simulink model "mcb_pmsm_sixstep_hall_dsPIC33CK256MP508"  (R2022a)
settings: Solver=FixedStepDiscrete  StartTime=0.0  StopTime=12  FixedStep=.00005  RelTol=1e-3  EnableMultiTasking=on
PreLoadFcn:
  | mcb_pmsm_sixstep_hall_lvmc_data;
InitFcn:
  | mcb_pmsm_sixstep_hall_lvmc_data;
values from neighbouring files (symbols this model uses):
  PI_params = mcb.internal.SetControllerParameters(bldc,inverter,PU_System,T_pwm,Ts,Ts_speed)    [mcb_bldc_sixstep_hall_lvmc_data.m]    (also in mcb_pmsm_sixstep_hall_lvmc_data.m)
  PU_System = mcb_SetPUSystem(bldc,inverter)    [mcb_bldc_sixstep_hall_lvmc_data.m]    (also in mcb_pmsm_sixstep_hall_lvmc_data.m)
  PWM_frequency = 20e3    (= 20000)    [mcb_bldc_sixstep_hall_lvmc_data.m]    (also in mcb_pmsm_sixstep_hall_lvmc_data.m)
  Ts = T_pwm    (= 5e-05)    [mcb_bldc_sixstep_hall_lvmc_data.m]    (also in mcb_pmsm_sixstep_hall_lvmc_data.m)
  Ts_speed = 30*Ts    (= 0.0015)    [mcb_bldc_sixstep_hall_lvmc_data.m]    (also in mcb_pmsm_sixstep_hall_lvmc_data.m)
undefined symbols (not defined in the file or in its folder): A0, AN0, AN1, B0, B2, bldc, C9, D13, inverter, MaxPer, ms, P32, P57, P77, Pin, pmsm, PWM1max, Resol, s, us
libraries: MCHP_Blockset x22, nesl_utility x14, simulink x12, fl_lib x9, ee_lib x5, mcbcontrolslib x4, mcbpositiondecoderlib x2, slpidlib x1
(part 1 of 3)
settings Model: Creator=M91449  LastModifiedBy=I52209
settings SolverCC: AlgebraicLoopSolver=TrustRegion
settings DataIOCC: LimitDataPoints=on  ReturnWorkspaceOutputs=off
settings OptimizationCC: DefaultParameterBehavior=Inlined  InlineInvariantSignals=on  LifeSpan=1  EfficientTunableParamExpr=on
settings DebuggingCC: MultiTaskDSMMsg=none  UnconnectedInputMsg=warning  UnconnectedOutputMsg=warning  UnconnectedLineMsg=warning  SFUnexpectedBacktrackingDiag=warning  SFNoUnconditionalDefaultTransitionDiag=warning  SFExecutionAtInitializationDiag=none  SFMachineParentedDataDiag=warning  ArithmeticOperatorsInVariantConditions=warning
settings HardwareCC: ProdBitPerInt=16  ProdBitPerPointer=16  ProdBitPerSizeT=16  ProdBitPerPtrDiffT=16  ProdLargestAtomicInteger=Integer  ProdLargestAtomicFloat=None  ProdWordSize=16  ProdHWDeviceType=Generic->Custom
settings ModelReferenceCC: ModelReferenceNumInstancesAllowed=Single  PropagateSignalLabelsOutOfModel=off
settings SFSimCC: SimUseLocalCustomCode=off  MATLABDynamicMemAlloc=off  CustomCodeUndefinedFunction=UseInterfaceOnly
settings RTWCC: Description=Microchip Embedded Target PIC24 dsPIC30 dsPIC33 (real-time)  SystemTargetFile=MCHP_dsPIC_stf.tlc  TemplateMakefile=MCHP_dsPIC.tmf  RTWUseLocalCustomCode=off  CustomInclude=/Clib  CustomSource=function.c  IncludeHyperlinkInReport=on  GenerateCodeMetricsReport=on  DLArmComputeVersion=19.05
settings CodeAppCC: IgnoreCustomStorageClasses=off  MaxIdLength=255  StateflowObjectComments=on
settings STFCustomTargetCC: TargetLibSuffix=_lib.a  CodeReplacementLibrary=Microchip Code Replacement Library for dsPIC  CombineOutputUpdateFcns=on  ERTCustomFileBanners=on  SupportContinuousTime=off  RemoveResetFunc=on  MATLABClassNameForMDSCustomization=Simulink.SoftwareTarget.ERTCustomization  GRTInterface=off  SystemTargetFile=MCHP_dsPIC_stf.tlc
settings ERTTargetCC: TargetLibSuffix=_lib.a  CodeReplacementLibrary=Microchip Code Replacement Library for dsPIC  MultiwordLength=2048  ParMdlRefBuildCompliant=off  CompOptLevelCompliant=off  ConcurrentExecutionCompliant=off  SupportNonInlinedSFcns=on  ModelStepFunctionPrototypeControlCompliant=off  CPPClassGenCompliant=off  UseToolchainInfoCompliant=off  InlinedParameterPlacement=NonHierarchical  ERTSrcFileBannerTemplate=MCHP_dsPIC_code_template.cgt  ERTHdrFileBannerTemplate=MCHP_dsPIC_code_template.cgt  ERTDataSrcFileTemplate=MCHP_dsPIC_code_template.cgt  ERTDataHdrFileTemplate=MCHP_dsPIC_code_template.cgt  ERTCustomFileTemplate=MCHP_main.tlc  ConvertIfToSwitch=off  SuppressUnreachableDefaultCases=off
settings ConfigComp: CovMetricSettings=dw  CovSaveCumulativeToWorkspaceVar=on  CovSaveSingleToWorkspaceVar=on  CovExternalEMLEnable=off

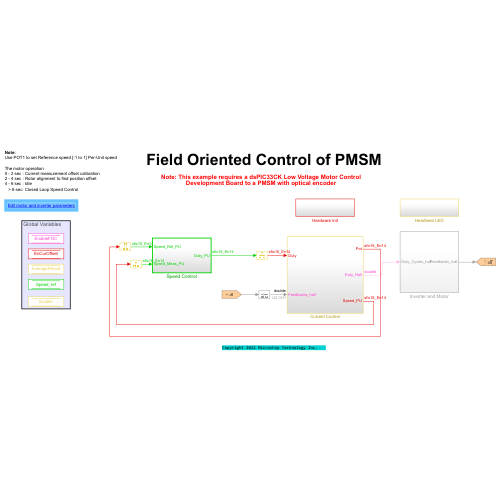
[thumbnail: Simulink's stored preview of the top-level diagram]
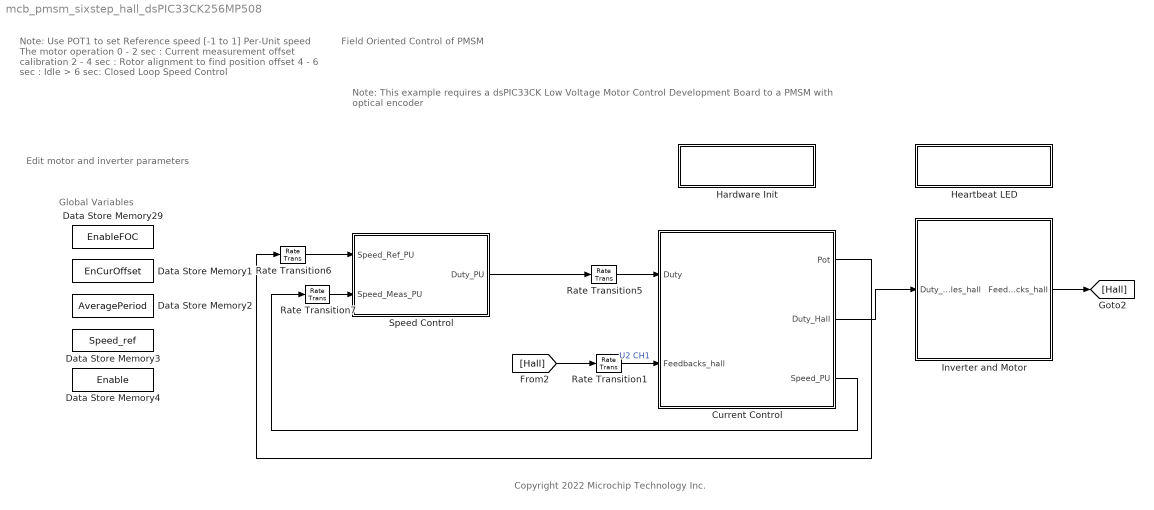
== system mcb_pmsm_sixstep_hall_dsPIC33CK256MP508 ==
  note: Edit motor and inverter parameters
  note: Note:
      | Use POT1 to set Reference speed [-1 to 1] Per-Unit speed
      |
      | The motor operation
      | 0 - 2 sec : Current measurement offset calibration
      | 2 - 4 sec : Rotor alignment to find position offset
      | 4 - 6 sec : Idle
      | > 6 sec: Closed Loop Speed Control
  note: Global Variables
  note: Field Oriented Control of PMSM
  note: Note: This example requires a dsPIC33CK Low Voltage Motor Control Development Board to a PMSM with optical encoder
  note: Copyright 2022 Microchip Technology Inc.
  Current Control : Subsystem  VariantControl=Optimized
  Data Store Memory1 : DataStoreMemory  DataStoreName=EnCurOffset  ShowAdditionalParam=off  OutDataTypeStr=boolean
  Data Store Memory2 : DataStoreMemory  DataStoreName=AveragePeriod  ShowAdditionalParam=off  OutDataTypeStr=uint16
  Data Store Memory29 : DataStoreMemory  DataStoreName=EnableFOC  ShowAdditionalParam=off  OutDataTypeStr=boolean
  Data Store Memory3 : DataStoreMemory  DataStoreName=Speed_ref  ShowAdditionalParam=off  OutDataTypeStr=dataType
  Data Store Memory4 : DataStoreMemory  DataStoreName=Enable  ShowAdditionalParam=off  OutDataTypeStr=boolean
  Hardware Init : Subsystem
  Heartbeat LED : Subsystem
  Inverter and Motor : Subsystem
  Rate Transition{1,5..7} (4 alike) : RateTransition  Deterministic=off
  Speed Control : Subsystem  TreatAsAtomicUnit=on  SystemSampleTime=Ts_speed
  wires:
  Rate Transition6/1 -> Speed Control/1(Speed_Ref_PU)
  Rate Transition7/1 -> Speed Control/2(Speed_Meas_PU)
  Speed Control/1(Duty_PU) -> Rate Transition5/1
  Rate Transition5/1 -> Current Control/1(Duty)
  Current Control/1(Pot) -> Rate Transition6/1
  Rate Transition1/1 -> Current Control/2(Feedbacks_hall)  "U2 CH1"
  Inverter and Motor/1(Feedbacks_hall) -> [Hall]
  [Hall] -> Rate Transition1/1
  Current Control/2(Duty_Hall) -> Inverter and Motor/1(Duty_Cycles_hall)
  Current Control/3(Speed_PU) -> Rate Transition7/1

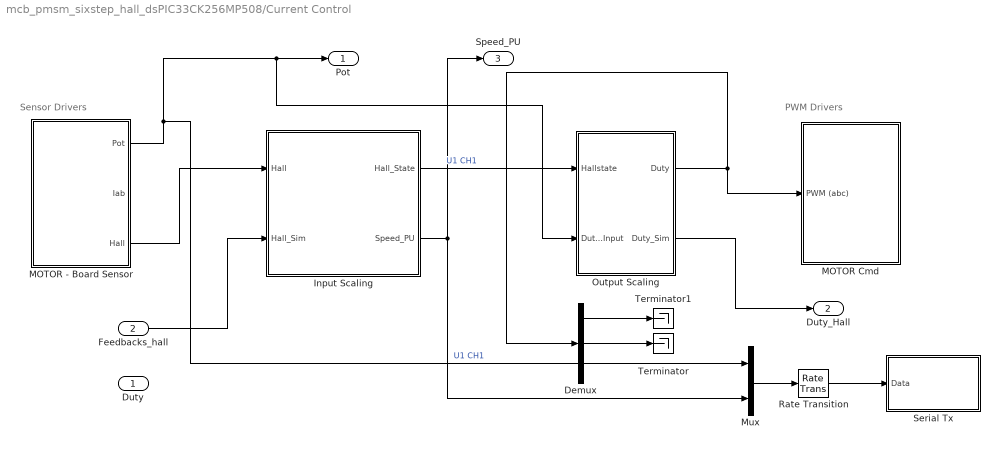
== system mcb_pmsm_sixstep_hall_dsPIC33CK256MP508/Current Control ==
  note: Sensor Drivers
  note: PWM Drivers
  Duty : Inport
  Feedbacks_hall : Inport  Port=2
  Demux : Demux  Outputs=3
  Input Scaling : Subsystem
  MOTOR Cmd : Subsystem
  MOTOR - Board Sensor : Subsystem
  Mux : Mux  Inputs=2
  Output Scaling : Subsystem
  Rate Transition : RateTransition  Integrity=off  Deterministic=off  OutPortSampleTime=Ts*100
  Serial Tx : Subsystem
  Terminator : Terminator
  Terminator1 : Terminator
  Pot : Outport
  Duty_Hall : Outport  Port=2
  Speed_PU : Outport  Port=3
  wires:
  Rate Transition/1 -> Serial Tx/1(Data)
  Mux/1 -> Rate Transition/1
  Feedbacks_hall/1 -> Input Scaling/2(Hall_Sim)
  Input Scaling/1(Hall_State) -> Output Scaling/1(Hallstate)  "U1 CH1"
  Output Scaling/1(Duty) -> MOTOR Cmd/1(PWM (abc)), Demux/1
  Output Scaling/2(Duty_Sim) -> Duty_Hall/1
  Demux/2 -> Terminator/1
  Demux/1 -> Terminator1/1
  MOTOR - Board Sensor/1(Pot) -> Mux/1, Output Scaling/2(Duty_Input), Pot/1  "U1 CH1"
  Input Scaling/2(Speed_PU) -> Mux/2, Speed_PU/1
  MOTOR - Board Sensor/3(Hall) -> Input Scaling/1(Hall)

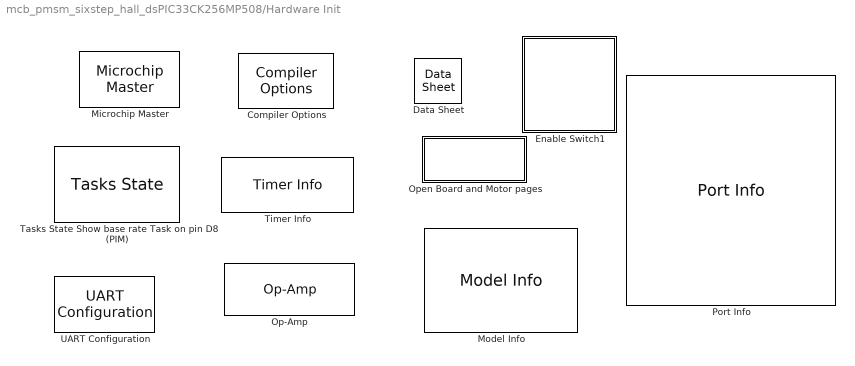
== system mcb_pmsm_sixstep_hall_dsPIC33CK256MP508/Hardware Init ==
  Compiler Options : MCHP_Blockset/System Configuration/Compiler Options  Priority=1  LATEST_CMPLR=on  COMP_LIST=Dynamic Options  COMP_LIST_TXT=xc16 - v1.70  DFP_LIST=Dynamic Options  DFP_LIST_TXT=v 1.7.208  CMSIS_DSP=Dynamic Options  CMSIS_DSP_TXT=Dynamic Options  USE_64BIT_DOUBLE=off  MCHP_MULTITHREAD_COMPILATION=on  UseCustom_LinkerScript=off  MCHP_MASTERLINK=mcb_pmsm_sixstep_hall_dsPIC33CK256MP508/Hardware Init/Microchip Master  OPTIMIZATION_LEVEL=3  MPLAB_LINKLIB=default  MPLAB_LINKLIB1=default  CodeReplacement=Dynamic Options  CodeReplacement_TXT=Microchip Code Replacement Library for dsPIC  OPTIMIZATION_FLTO=on  OPTIMIZATION_REORDER=off  UNROLL_LOOPS=on  PROCEDURAL_ABSTRACTION=off  MCODE=is less than 32768 (faster)  MCONST=in data memory  MDATA=Use only memory below address 8192 (faster)  MSCALAR=Use only memory below address 8192 (faster)  MLARGEARRAY=off  MAGGREGATE=off  HEAP_SIZE=0  OMF=elf  DEBUG_INFO=off  ProduceHexOutput=on  AssemblyListing=off  SaveTemps=off  NO_EDS_WARN=on  PRINT_STATISTICS=off
      settings: SourceProductName=MPLAB Device Blocks for Simulink
  Data Sheet : MCHP_Blockset/System Info/Data Sheet  DOC_Type=datasheet  DOC_MCHP_Id=33CK256MP508_datasheet  DOC_FilePath=C:\Users\M91449\AppData\Local\Temp\dsPIC33CK256MP508-Family-Data-Sheet-DS70005349F.pdf  DOC_FileLastCheckTime="[2019              4             12             18             23         53.807]"  cpy_MCHP_Id=33CK256MP508  MCHP_MASTERLINK=mcb_pmsm_sixstep_hall_dsPIC33CK256MP508/Hardware Init/Microchip Master
      settings: AttributesFormatString=%<cpy_MCHP_Id>  SourceProductName=MPLAB Device Blocks for Simulink
  Enable Switch1 : Subsystem  Variant=on  VariantControlMode=sim codegen switching
  Microchip Master : MCHP_Blockset/System Configuration/Microchip Master  Priority=1  PICREF=33CK256MP508  TIMESTEP_REF=PWM1 Trigger 1 + ADC  BUSYFLAG=Dynamic Options  BUSYFLAG_TXT=None  VDD_range=Dynamic Options  PWRTEN=Not used  BOREN=Disable  BODENV=2.7V  BORV=Not used  FPWRT=128ms  DSBOREN=Enable ZPBOR during Deep Sleep Mode  DSLPBOR=Not used  MCLRE=Enabled  SMCLR=MCLR pin generates a normal system Reset  PMDL1WAY=Allow only one reconfiguration  RSTPRI=Device will obtain reset instruction from Primary flash  TEMP=Not used  SOSCSRC=Not used  SOSCSEL=Not used  IOL1WAY=Allow only one reconfiguration  ALTVREF=Not used  DISUVREG=Not used  DSSWEN=Not used  LPCFG=Not used  RTCBAT=Not used  VBTBOR=Not used  WUTSEL=Not used  POWERSAVE=off  FNOSC=Internal Fast RC (FRC)  FPR=ECIO w/ PLL 16x  FOSFPR=HS3 w/PLL 16x  FOS=Primary Oscillator  FRANGE=High Range  OSCILLATOR_SELECT=Internal Fast RC (FRC)  OSCILLATOR_SELECT_spd=Internal Fast RC (FRC)  QUARTZ=8e6  QUARTZ_spd=8e6  POSCGAIN=2x gain setting  POSCBOOST=Boost the kick start of the oscillator  SOSCGAIN=2x gain setting  SOSCBOOST=Boost the kick start of the oscillator  ACTIV_PLL=on  ACTIV_PLL_spd=on  MIPS_DESIRED=100e6  MIPS_DESIRED_spd=100e6  CPUDIV=Divide by 1  FPLLMUL=Not used  FPLLIDIV=8x Divider  POSCFREQ=Not used  POSCMD=Primary Oscillator Disabled  POSCMOD=Primary Oscillator Disabled  MIPS=100 * 1e6  ACLKCON=Optimized for PWM resolution & ADC conversion speed  ACLKCON_spd=Optimized for PWM resolution & ADC conversion speed  FPLLODIV=32x Divider  PLLKEN=PLL lock signal will be used to disable PLL clock output if lock is lost  FCKSM=Clock switching is enabled;Fail-safe Clock Monitor is disabled  FCKSMEN=Sw Disabled; Mon Disabled  IESO=Start up with FRC; then switch  DSWDTPS=1:2^36  FWDTEN=WDT controlled via SW; use WDTCON.ON bit  FWDTWINSZ=Window size is 25%  FWPSA=1:512  FWPSA0=1:128  FWPSB=1:16  WDT=Disable  WDTPOST=1:32768  WDTPRE=1:128  WDTPS=1:32768  WINDIS=Watchdog Timer operates in Non-Window mode  WWDTEN=Non-Window mode  DSWDTEN=Enable DSWDT during Deep Sleep Mode  DSWDTOSC=Select LPRC as DSWDT Reference clock  FPBDIV=Not used  FSOSCEN=Disable Secondary Oscillator  LPRCSEL=Not used  OSCIOFCN=Not used  OSCIOFNC=general purpose digital I/O pin  LVRCFG=Not used  PLL_96MHZ=Not used  PLL96MHZ=Not used  PLLDIV=Not used  WDTCLK=Not used  WDTCMX=Not used  WDTWIN=WDT Window is 25% of WDT period  XTCFG=24-32 MHz crystals  XTBST=Boost the kick-start  APL=Aux Flash Code protect is disabled  APLK=Aux Flash Write Protection or Code Protection is Enabled  AWRP=Auxiliary program memory is not write-protected  BSS=No Protection (other than BWRP)  BWP=Not used  BWRP=Boot Segment may be written  CP=Protection Disabled  EBS=No Boot EEPROM  ESS=No Segment Data EEPROM  GCP=General Segment Code protect is Disabled  GSS=No Protection (other than GWRP)  GSS0=Not used  GSSK=General Segment Write Protection or Code Protection is Enabled  GWRP=General Segment may be written  PWP=Not used  RBS=No Boot RAM  RSS=No Secure RAM  SSS=No Secure Segment  SWRP=Secure segment may be written  WPCFG=Not used  WPDIS=Not used  WPEND=Not used  WPFP=Not used  ICESEL=Communicate on PGEC1/PGED1  ICS=Communicate on PGC3 and PGD3  JTAGEN=Disable  COE=Not used  RES=Not used  DEBUG=Debugger is disabled  BACKBUG=Not used  BKBUG=Not used  ALTI2C=I2C mapped to SDA1/SCL1 pins  ALTI2C1=I2C1 mapped to SDA1/SCL1 pins  ALTI2C2=I2C2 mapped to SDA2/SCL2 pins  ALTI2C3=I2C3 mapped to SDA3/SCL3 pins  ALTQIO=QEA1; QEB1; INDX1 are selected as inputs to QEI1  ALTSS1=SS1A is selected as the I/O pin for SPI1  CMPPOL0=Hysteresis is applied to falling edge  CMPPOL1=Hysteresis is applied to falling edge  FCANIO=Not used  FETHIO=Default Ethernet I/O  FMIIEN=MII Enabled  FSRSSEL=Not used  FUSBIDIO=Controlled by the USB Module  FVBUSONIO=Not used  HPOL=PWM module high side output pins have active-high output polarity  HYST0=45 mV Hysteresis  HYST1=45 mV Hysteresis  I2C1SEL=Not used  LPOL=PWM module low side output pins have active-high output polarity  PWMPIN=PWM module pins controlled by PORT register at device Reset  RTCOSC=Not used  UPLLEN=USB PLL Disabled  UPLLIDIV=Not used  ATMOD8=Not used  ALTPMP=Not used  I2C2SEL=Not used  ALTADREF=Not used  ALTCVREF=Not used  PWMLOCK=PWM registers may be written without key sequence  INT_PRIORITY_DMA=0  MCHP_TIMER_RESULT=[ ]  MCHP_PLLRegisters="[1    100  16387     -1     33]"  MCHPVAR=MCHP.fcy.MIPS=1e+08;MCHP.fcy.SYSCLK=1e+08;MCHP.fcy.ADC=1e+08;MCHP.fcy.Comparator=1e+08;MCHP.fcy.I2C=1e+08;MCHP.fcy.SPI=1e+08;MCHP.fcy.UART=2e+08;MCHP.fcy.Timers=1e+08;MCHP.fcy.OC=1e+08;MCHP.fcy.IC=1e+08;MCHP.fcy.Ports=1e+08;MCHP.fcy.QEI=1e+08;MCHP.fcy.APLL=-1;MCHP.PowerSave=0;MCHP.TimeStepFactor=-20000;MCHP.TimeStep_Timer=-1;MCHP.NTIMERS=1;MCHP.id.name='33CK256MP508';MCHP.id.N=reshape([33 256 508],1,3);MCHP.id.L=reshape({ 'CK','MP',''},1,3);MCHP.id.Arch=3;MCHP.periph.PPS.reg_RPINRx=reshape([-1 1 1 1 -1 1 1 1 1 1 1 1 1 1 1 1 1 1 1 1 1 1 -1 -1 1 1 1 1 1 1 1 1 1 1 1 1 1 1 1 1 1 1 1 -1 1 1 1 -1 -1 -1 -1 -1 1 -1 1 1 -1 -1 1 1 1 -1 -1 -1 -1 1 1 -1 -1 -1 -1 -1 -1 -1 -1 1 1 -1 -1 -1 -1 -1 -1 -1 1 1 1 1 1 1 1 -1 -1 -1 -1 -1 -1 1 1 1],1,100);MCHP.PPS.dsPIC.RP=reshape([-1 -1 -1 -1 -1 -1 -1 -1 -1 -1 -1 -1 -1 -1 -1 -1 -1 -1 -1 -1 -1 -1 -1 -1 -1 -1 -1 -1 -1 -1 -1 -1 16 17 18 19 20 21 22 23 24 25 26 27 28 29 30 31 32 32 33 35 36 37 38 34 40 41 42 43 44 45 46 47 48 49 50 51 52 53 54 55 56 57 35 59 60 61 62 63],1,80);MCHP.PPS.dsPIC.RPI=reshape(MCHP_Fun.Hex2num('[]'),0,0);MCHP.PPS.dsPIC.RPINR_list=reshape({ '1','INT1','INT2','INT3','5','T1CK','TCKI1','ICM1','TCKI2','ICM2','TCKI3','ICM3','TCKI4','ICM4','TCKI5','ICM5','TCKI6','ICM6','TCKI7','ICM7','TCKI8','ICM8','OCFA','OCFB','PCI8','PCI9','PCI10','PCI11','QEIA1','QEIB1','QEINDX1','QEIHOM1','QEIA2','QEIB2','QEINDX2','QEIHOM2','U1RX','U1DSR','U2RX','U2DSR','SDI1','SCK1_in','SS1_in','REFOI','SDI2','SCK2_in','SS2_in','48','49','50','51','52','CAN1RX','54','U3RX','U3DSR','57','58','SDI3','SCK3_in','SS3_in','62','63','64','65','TCKI9','ICM9','68','69','70','71','72','73','74','OCFC','PCI17','PCI18','78','79','80','81','82','83','84','PCI12','PCI13','PCI14','PCI15','PCI16','SENT1','SENT2','CLCINA','CLCINB','CLCINC','CLCIND','ADCTRG','OCFD','U1CTS','U2CTS','U3CTS'},1,100);MCHP.PPS.dsPIC.RPOR_list=reshape({ '1','U1TX','U1RTS','U2TX','U2RTS','SDO1','SCK1_out','SS1_out','SDO2','SCK2_out','SS2_out','SDO3','SCK3_out','SS3_out','REFCLKO','OCM1','OCM2','OCM3','OCM4','OCM5','OCM6','CAN1','22','CMP1','CMP2','CMP3','26','U3TX','U3RTS','29','30','31','32','33','PWM4H','PWM4L','PWMEA','PWMEB','QEICCMP1','QEICCMP2','CLC1OUT','CLC2OUT','OCM7','OCM8','PWMEC','PWMED','PTGTRG24','PTGTRG25','SENT1OUT','SENT2OUT','MCCP9A','MCCP9B','MCCP9C','MCCP9D','MCCP9E','MCCP9F','56','57','58','CLC3OUT','CLC4OUT','U1DTR','U2DTR','U3DTR'},1,64);MCHP.PPS.map_RPnR_RPORx=reshape([32 33 34 35 36 37 38 39 40 41 42 43 44 45 46 47 48 49 50 51 52 53 54 55 56 57 58 59 60 61 62 63 64 65 66 67 68 69 70 71 72 73 74 75 76 77 78 79 176 177 178 179 180 181],1,54);MCHP.Rx=reshape([16 34 15 74 2 -1 -1 -1 -1 -1 -1 18 35 28 73 4 -1 -1 -1 -1 -1 -1 20 41 29 72 17 -1 -1 -1 -1 -1 -1 21 43 33 69 19 -1 -1 -1 -1 -1 -1 23 45 63 68 22 -1 -1 -1 -1 -1 -1 -1 55 65 54 24 -1 -1 -1 -1 -1 -1 -1 56 30 53 37 -1 -1 -1 -1 -1 -1 -1 58 40 52 39 -1 -1 -1 -1 -1 -1 -1 60 46 49 42 -1 -1 -1 -1 -1 -1 -1 61 47 48 44 -1 -1 -1 -1 -1 -1 -1 75 66 38 57 -1 -1 -1 -1 -1 -1 -1 76 67 36 59 -1 -1 -1 -1 -1 -1 -1 78 5 27 62 -1 -1 -1 -1 -1 -1 -1 80 6 14 64 -1 -1 -1 -1 -1 -1 -1 1 7 13 77 -1 -1 -1 -1 -1 -1 -1 3 8 10 79 -1 -1 -1 -1 -1 -1],11,16);MCHP.ADC.ANtype=reshape([0 0],1,2);MCHP.ADC.ADCONx=reshape([0 0 0 0 0 0],1,6);MCHP.ADC.ADCHS_0=reshape([0 0],1,2);MCHP.ADC.Flags=reshape([-1 0],1,2);MCHP.ADC.Buffer=reshape([-1 -1],1,2);MCHP.ADC.port=reshape([0 18 23 3 4 16 17 -1 19 2 24 25 32 33 34 35 39 38 58 59 64 65 66 67 -1 -1 -1 -1 -1 -1 -1 -1 -1 -1 -1 -1 -1 -1 -1 -1 -1 -1 -1 -1 -1 -1 -1 -1 -1 -1 -1 -1 -1 -1 -1 -1 -1],1,57);MCHP.ADC.port_ALT=reshape([18 1 -1 -1],1,4);MCHP.ADC.port_VrefP=-1;MCHP.ADC.port_VrefM=-1;MCHP.ADC.port_AVdd=-1;MCHP.ADC.port_AVss=-1;MCHP.ADC.ADCDATA=reshape([1 1 1 1 1 1 1 1 1 1 1 1 1 1 1 1 1 1 1 1 1 1 1 1 1 1 0 0 0 0 0 0 0 0 0 0 0 0 0 0 0 0 0 0 0 0 0 0 0 0 0 0 0 0 0 0 0],1,57);MCHP.ADC.HS_SAR.TRGSRC=reshape([1 1 1 1 1 1 1 1 1 1 1 1 1 1 1 1 1 1 1 1 1 1 1 1 1 1 0 0 0 0 0 0],1,32);MCHP.ADC.HS_SAR.nFilters=4;MCHP.ADC.HS_SAR.nDedicatedCore=2;MCHP.ADC.HS_SAR.CALIBRATION=0;MCHP.ADC.HS_SAR.ADCON1L=40960;MCHP.ADC.HS_SAR.ADC_Class3_idxStart=26;MCHP.memory.RAM=24576;MCHP.memory.RAM_XBegin=4096;MCHP.memory.RAM_YBegin=20480;MCHP.memory.RAM_dma=reshape([-1 -1],1,2);MCHP.memory.FLASH_ECC=0;MCHP.DMA.Num=0;MCHP.DMA.CNTmax=0;MCHP.QEI.QEICONx=reshape([49023 49023 -1 -1 -1 -1],1,6);MCHP.QEI.QEItype=2;MCHP.QEI.Port_QEI_INDX=reshape([-1 -1],1,2);MCHP.QEI.Port_QEI_QEA=reshape([-1 -1],1,2);MCHP.QEI.Port_QEI_QEB=reshape([-1 -1],1,2);MCHP.QEI.Port_QEI_UPDN=reshape([-1 -1],1,2);MCHP.INT.Port=reshape([18 32767 32767 32767 -1],1,5);MCHP.PWM_HS.Flags=reshape([0 0 0],1,3);MCHP.PWM.port_FLT=reshape([-1 -1 -1 -1 -1 -1 -1 -1 -1 -1 -1 -1 -1 -1 -1 -1 -1 -1 -1 -1 -1 -1 -1 -1 -1 -1 -1 -1 -1 -1 -1 -1 -1],1,33);MCHP.PWM.PWMRef=-1;MCHP.PWM.Flag=0;MCHP.PWM.Port_PWM_l=reshape([31 -1 29 -1 27 -1 48 -1 37 -1 47 -1 43 -1 45 -1 -1 -1 -1 -1 -1 -1 -1 -1],2,12);MCHP.PWM.Port_PWM_h=reshape([30 -1 28 -1 26 -1 49 -1 36 -1 46 -1 42 -1 44 -1 -1 -1 -1 -1 -1 -1 -1 -1],2,12);MCHP.PWM_HS_FEP.nEVTOUT=5;MCHP.IC.Port=reshape([0 0 0 0 0 0 0 0 0 0 0 0 0 0 0 0],1,16);MCHP.IC.type=-1;MCHP.OC.Port=reshape([0 0 0 0 0 0 0 0 0 0 0 0 0 0 0 0],1,16);MCHP.OC.type=-1;MCHP.CN.Port=reshape([-1 -1 -1 -1 -1 -1 -1 -1 -1 -1 -1 -1 -1 -1 -1 -1 -1 -1 -1 -1 -1 -1 -1 -1 -1 -1 -1 -1 -1 -1 -1 -1 -1 -1 -1 -1 -1 -1 -1 -1 -1 -1 -1 -1 -1 -1 -1 -1 -1 -1 -1 -1 -1 -1 -1 -1 -1 -1 -1 -1 -1 -1 -1 -1 -1 -1 -1 -1 -1 -1 -1 -1 -1 -1 -1 -1 -1 -1 -1 -1 -1 -1 -1 -1 -1],1,85);MCHP.CN.PullUp=reshape([31 65535 65535 65535 65535 0 0 0 0 0 0],1,11);MCHP.CN.type=2;MCHP.CN.Flag_PullDown=1;MCHP.SPI.Refs=reshape([1 2 3 0 0 0],1,6);MCHP.SPI.SPIxCON1=-1;MCHP.SPI.SPIxCON2=-1;MCHP.SPI.Port_SDI=reshape([-1 41 -1 -1 -1 -1],1,6);MCHP.SPI.Port_SDO=reshape([-1 56 -1 -1 -1 -1],1,6);MCHP.SPI.Port_SCK=reshape([-1 40 -1 -1 -1 -1],1,6);MCHP.SPI.Port_SS=reshape([-1 -1 -1 -1 -1 -1],1,6);MCHP.I2C.Refs=reshape([1 2 3 0 0],1,5);MCHP.I2C.I2CxCON=49151;MCHP.I2C.NewRegName=2;MCHP.I2C.Port_SDA=reshape([25 21 23 -1 -1],1,5);MCHP.I2C.Port_SCL=reshape([24 22 18 -1 -1],1,5);MCHP.I2C.Port_ASDA=reshape([40 36 52 -1 -1],1,5);MCHP.I2C.Port_ASCL=reshape([41 37 51 -1 -1],1,5);MCHP.I2C.Fuse_Port_SCL_SDA=reshape([27 1 28 1 29 1 -1 -1 -1 -1],2,5);MCHP.I2C.Fuse_Port_ASCL_ASDA=reshape([27 2 28 2 29 2 -1 -1 -1 -1],2,5);MCHP.SCCP.nSCCP=9;MCHP.SCCP.MCCP=reshape([0 0 0 0 0 0 0 0 1],1,9);MCHP.PGA.Port_PGA1P=reshape([-1 -1 -1 -1],1,4);MCHP.PGA.Port_PGA1N=reshape([-1 -1 -1 -1],1,4);MCHP.PGA.Port_PGA2P=reshape([-1 -1 -1 -1],1,4);MCHP.PGA.Port_PGA2N=reshape([-1 -1 -1 -1],1,4);MCHP.PGA.Num=0;MCHP.HS_AnalogComparator.Port_CMP1=reshape([0 33 3 18],1,4);MCHP.HS_AnalogComparator.Port_CMP2=reshape([35 34 59 18],1,4);MCHP.HS_AnalogComparator.Port_CMP3=reshape([23 4 58 18],1,4);MCHP.HS_AnalogComparator.Port_CMP4=reshape([-1 -1 -1 -1],1,4);MCHP.HS_AnalogComparator.PORT_EXTREFx=reshape([-1 -1],1,2);MCHP.HS_AnalogComparator.Port_DACOUTx=reshape([3 -1],1,2);MCHP.HS_AnalogComparator.Num=0;MCHP.Comp.Port_CVrefin=-1;MCHP.Comp.Port_CVref=-1;MCHP.Comp.Port_CVref1O=-1;MCHP.Comp.Port_CVref2O=-1;MCHP.Comp.Port_CxOUT=reshape([32767 32767 32767 32767 32767],1,5);MCHP.Comp.Port_OAxOUT=reshape([0 18 4 -1 -1],1,5);MCHP.Comp.Port_CxINP=reshape([-1 -1 -1 -1 -1],1,5);MCHP.Comp.Port_CxINM=reshape([-1 -1 -1 -1 -1 -1 -1 -1 -1 -1 -1 -1 -1 -1 -1 -1 -1 -1 -1 -1],4,5);MCHP.Comp.Port_OAxINP=reshape([2 20 34 -1 -1],1,5);MCHP.Comp.Port_OAxINM=reshape([1 19 33 -1 -1],1,5);MCHP.Comp.nComp=reshape([5 0 0],1,3);MCHP.Comp.OpAmp=0;MCHP.Comp.CVRCON=reshape([0 0],1,2);MCHP.Comp.CMCON=0;MCHP.CDAC.Port_DACx=reshape([-1 -1 -1],1,3);MCHP.CDAC.nCDAC=0;MCHP.UART.port_Rx=reshape([32767 32767 32767 -1 -1 -1],1,6);MCHP.UART.port_Tx=reshape([32767 32767 32767 -1 -1 -1],1,6);MCHP.UART.port_ARx=reshape([-1 -1],1,2);MCHP.UART.port_ATx=reshape([-1 -1],1,2);MCHP.UART.port_RTS=reshape([32767 32767 32767 -1 -1 -1],1,6);MCHP.UART.port_CTS=reshape([32767 32767 32767 -1 -1 -1],1,6);MCHP.UART.reg_UxMODE=reshape([48127 48127 48127 -1 -1 -1],1,6);MCHP.UART.reg_UxSTA=reshape([65535 65535 65535 -1 -1 -1],1,6);MCHP.modsrc.DOS_02551_cpu_16bit_v7=1;MCHP.modsrc.DOS_01520_wdt_dmt_upb_v1_16bit=1;MCHP.modsrc.DOS_02359a_sent_j2716_upb_v1=1;MCHP.modsrc.DOS_02672_math_progcrc_upb_v1_16bit=1;MCHP.modsrc.DOS_01577_cla_clc_upb_v1=1;MCHP.modsrc.DOS_02915_ecc_v2=1;MCHP.modsrc.DOS_02673_tmr_classa_upb_v1_16bit=1;MCHP.modsrc.DOS_01494_qei_32b_upb_v1_16bit=1;MCHP.modsrc.DOS_02552_msi_upb_v1_Master=0;MCHP.modsrc.DOS_01441_i2c_upb_v1_16bit_TLAH=1;MCHP.modsrc.DOS_03076_uart_protocol_upb_v1_16bit=1;MCHP.modsrc.DOS_01482=1;MCHP.modsrc.DOS_03667_pwm_pc_upb_v2_16bit=0;MCHP.modsrc.DOS_03247_CAN_FD_UPB_V2_16_bit=1;MCHP.modsrc.DOS_04180_drm_ctrl_ecc_v1=0;MCHP.modsrc.DOS_03431_STX03=0;MCHP.modsrc.DOS_02316_nvm_ctrl_v1_16bit=1;MCHP.modsrc.DOS_01459_ptg_pc_upb_v1_16bit=1;MCHP.modsrc.DOS_01512_ccp_mccp_upb_v1_16bit=1;MCHP.modsrc.DOS_02519_dma_sfr_16bit_v2=1;MCHP.modsrc.DOS_02508c11=1;MCHP.modsrc.DOS_02475_dac_pdm_nbit_upb_v1_16bit=1;MCHP.modsrc.DOS_03516_pwr_sib_upb_v3=0;MCHP.modsrc.DOS_02467_gpio_upb_v1_16bit=1;MCHP.modsrc.DOS_00805_rst_integration_v4=1;MCHP.modsrc.DOS_02659_clk_sib_v12=1;MCHP.modsrc.DOS_02674_wdt_upb_v1_16bit=1;MCHP.modsrc.DOS_01407=1;MCHP.modsrc.DOS_02552_msi_upb_v1_Slave=0;MCHP.modsrc.DOS_02593_amp_pga_ctrl_pb_v2_16bit=0;MCHP.modsrc.DOS_01483_pwm_16bit=1;MCHP.modsrc.DOS_02497_WACV=0;MCHP.modsrc.DOS_02653_afe_current_bias_ctrl_upb_v1_16bit=1;MCHP.modsrc.DOS_01461_afe_ctmu_con_upb_v1_16bit=0;MCHP.modsrc.DOS_02497_WACA=0;MCHP.modsrc.DOS_02478_uart_irda_upb_v1_16bit=0;MCHP.modsrc.DOS_00929=0;MCHP.modsrc.DOS_01198=0;MCHP.modsrc.DOS_03029_WACH=0;MCHP.modsrc.DOS_02472_ppi_pmp16_upb_v1_16bit=1;MCHP.modsrc.DOS_01483_apwm_16bit=0;MCHP.modsrc.DOS_04797_WAC0A=0;MCHP.modsrc.DOS_03349_amp_pad_opamp_ctrl_upb_v1=1;MCHP.modsrc.DOS_02237_osc_dco_ctrl_upb_v1_16bit=1;MCHP.modsrc.DOS_04884_WAC0B=0;MCHP.modsrc.DOS_02949_WACG=1;MCHP.modsrc.DOS_04797_WAC09=0;MCHP.modsrc.DOS_03994_WAC07=0;MCHP.modsrc.DOS_03662_WACU=0;MCHP.modsrc.DOS_00794=0;MCHP.modsrc.DOS_00931=0;MCHP.modsrc.DOS_00932=0;MCHP.modsrc.DOS_00942=0;MCHP.modsrc.DOS_00938=0;MCHP.modsrc.DOS_00996=0;MCHP.modsrc.DOS_00997=0;MCHP.modsrc.DOS_00998=0;MCHP.modsrc.DOS_00209=0;MCHP.modsrc.DOS_01555_adc=0;MCHP.modsrc.DOS_01293=0;MCHP.modsrc.DOS_00828=0;MCHP.modsrc.DOS_01116=0;MCHP.modsrc.DOS_01017_RPORx=0;MCHP.modsrc.DOS_01017_RPINRx=0;MCHP.modsrc.DOS_01555_nvm_tsmc18_v2_16bit=0;MCHP.modsrc.DOS_00804=0;MCHP.modsrc.DOS_00826=0;MCHP.modsrc.DOS_01555_TLAK_PMDx=0;MCHP.modsrc.DOS_01555_TLAK_INT_=0;MCHP.modsrc.DOS_00933=0;MCHP.modsrc.DOS_01555=0;MCHP.modsrc.DOS_01555_ptg=0;MCHP.modsrc.DOS_00958=0;MCHP.modsrc.DOS_01117_PORTx=0;MCHP.modsrc.DOS_00999=0;MCHP.modsrc.DOS_01041=0;MCHP.modsrc.DOS_00892=0;MCHP.modsrc.DOS_01287_TLAC_PMDx=0;MCHP.modsrc.DOS_01287_TLAC_INT_=0;MCHP.modsrc.DOS_01424=0;MCHP.modsrc.DOS_01332=0;MCHP.modsrc.DOS_01468_PMBA_current_source=0;MCHP.modsrc.DOS_02291_PGA=0;MCHP.modsrc.DOS_01467_Comparator=0;MCHP.modsrc.DOS_01498_TLAY=0;MCHP.modsrc.DOS_00993_PLL_120MHz=0;MCHP.modsrc.DOS_01332_ptg_pc_v1=0;MCHP.modsrc.DOS_00958_pwm_TLAY=0;MCHP.modsrc.TLAY_IOPorts=0;MCHP.modsrc.DOS_00929q=0;MCHP.modsrc.DOS_02415_spi_v5=0;MCHP.modsrc.DOS_RPINRx_16bit_2=0;MCHP.modsrc.DOS_01497_TLAH_PMDx=0;MCHP.modsrc.DOS_02550_TLAL_INT=0;MCHP.modsrc.DOS_00958_pwm_TLAH=0;MCHP.modsrc.DOS_01287_TLAH_INT_=0;MCHP.modsrc.DOS_01113=0;MCHP.modsrc.DOS_01017_PMDx=0;MCHP.modsrc.DOS_00927=0;MCHP.modsrc.DOS_01080=0;MCHP.modsrc.DOS_00794_cpu_16bit_v3=0;MCHP.modsrc.DOS_02192_TLCD_PMDx=0;MCHP.modsrc.DOS_02192_TLCD_INT_=0;MCHP.modsrc.DOS_02192_cmp=0;MCHP.modsrc.DOS_00958_pwm_TLCD=0;MCHP.modsrc.DOS_02192_PORTx_TLCD=0;MCHP.modsrc.DOS_00936=0;MCHP.modsrc.DOS_00995=0;MCHP.modsrc.DOS_00546=0;MCHP.modsrc.DOS_00474=0;MCHP.modsrc.DOS_02481_WACK_MC_Config=0;MCHP.modsrc.DOS_03088_pfm_cache_ocp_v2_WACK=0;MCHP.modsrc.DOS_02819_pfm_ctrl_32bit_upb_v2=0;MCHP.modsrc.DOS_02674_wdt_upb_v1_32bit=0;MCHP.modsrc.DOS_01520_wdt_dmt_upb_v1=0;MCHP.modsrc.DOS_02869_icd_jtag_bvci_upb_v2=0;MCHP.modsrc.DOS_02823_WACJ_clk_cru_upb_v2=0;MCHP.modsrc.DOS_02823_WACN_clk_cru_upb_v2=0;MCHP.modsrc.DOS_01423_RPINRx=0;MCHP.modsrc.DOS_02481_RPORx=0;MCHP.modsrc.DOS_02511_pwr_sib_upb_v1_32bit=0;MCHP.modsrc.DOS_02907_WACN_GP_int_evic_v3=0;MCHP.modsrc.DOS_01500_dma_bvci_v2=0;MCHP.modsrc.DOS_02141_tmr_classa_pb_v2=0;MCHP.modsrc.DOS_02815_tmr_classb_upb_v1=0;MCHP.modsrc.DOS_00740_icap_pb_v1=0;MCHP.modsrc.DOS_00749_ocmp_pb_v1=0;MCHP.modsrc.DOS_01441_i2c_upb_v1_32bit=0;MCHP.modsrc.DOS_01329_spi_pb_v2=0;MCHP.modsrc.DOS_02478_uart_irda_upb_v1_32bit=0;MCHP.modsrc.DOS_03554_cmp_control_upb_v2_32bit=0;MCHP.modsrc.DOS_01445_dac_nbit__control_upb_v1_32bit=0;MCHP.modsrc.DOS_01461_afe_ctmu_con_upb_v1=0;MCHP.modsrc.DOS_01577_cla_clc_upb_v1_32bit=0;MCHP.modsrc.DOS_02467_gpio_ports_upb_v1=0;MCHP.modsrc.DOS_02508_adc_sar_ctrl_upb_v1_PIC32MK=0;MCHP.modsrc.DOS_01261_tmr_rtcc_pb_v2=0;MCHP.modsrc.DOS_01475_lpwr_deep_sleep_ctrl_v2=0;MCHP.modsrc.DOS_EIP_00136_ssx_v1=0;MCHP.modsrc.DOS_02907_WACN_MC_int_evic_v3=0;MCHP.modsrc.DOS_01477_pwm_mc_upb_v1=0;MCHP.modsrc.DOS_01494_qei_32b_upb_v1=0;MCHP.modsrc.DOS_03247_can_fd_upb_v2_pic32mk=0;MCHP.modsrc.DOS_02907_WACK_MC_int_evic_v3=0;MCHP.modsrc.DOS_02514_dfm_strl_sst_upb_v1=0;MCHP.modsrc.DOS_02472_ppi_pmp16_upb_v1=0;MCHP.modsrc.DOS_02813a_usb_otgcore_pb_v3=0;MCHP.modsrc.DOS_02481_WACJ_MC_Config=0;MCHP.modsrc.DOS_02569_pfm_cache_ocp_v1=0;MCHP.modsrc.DOS_02481_WACJ_MC_int_evic_v3=0;MCHP.modsrc.DOS_01459_ptg_pc_upb_v1_SIC=0;MCHP.modsrc.DOS_01427_cmp_control_upb_v1_32bit=0;MCHP.modsrc.DOS_01152_can_bvci_v1=0;MCHP.modsrc.DOS_02787_WACD_Config=0;MCHP.modsrc.DOS_00800_dac_4bit_ctrl_pb_v1=0;MCHP.modsrc.DOS_01539_icd_jtag_pb_v2=0;MCHP.modsrc.DOS_02823_clk_cru_upb_v2=0;MCHP.modsrc.DOS_01423_RPORx=0;MCHP.modsrc.DOS_02907_WACD_int_evic_v3=0;MCHP.modsrc.DOS_00734_uart_irda_pb_v1=0;MCHP.modsrc.DOS_00687_tmr_classa_pb_v1=0;MCHP.modsrc.DOS_00745_tmr_classb_pb_v1=0;MCHP.modsrc.DOS_02508_adc_sar_ctrl_upb_v1=0;MCHP.modsrc.DOS_00866_cmp_control_pb_v2=0;MCHP.modsrc.DOS_01114_eth_bvci_v1=0;MCHP.modsrc.DOS_02831_usb_clk_rst_v2=0;MCHP.modsrc.DOS_01643_pfm_cache_ahb_v2=0;MCHP.modsrc.DOS_EIP_00206r5_sqi_v2=0;MCHP.modsrc.DOS_EIP_00124_usb_hs_otgcore_v1=0;MCHP.modsrc.DOS_EIP_00218_math_rng_ahbs_v2=0;MCHP.modsrc.DOS_EIP_00109_ebi_v1=0;MCHP.modsrc.DOS_EIP_00158_crypto_v1=0;MCHP.PortBase=16;MCHP.PortPrefixe='P';MCHP.clock.PBxDIV=-1;  MCHP_CRC=15913400  BTMODE=Not used  RES1=Not used  PLLSS=Not used  RES2=Not used  ALTCMPI=Not used  BOREN1=Not used  ALTRB6=Not used  RETCFG=Not used  DFMCY=Not used  BSS2=No Boot Segment  BSEN=No Boot Segment  CWRP=Configuration Segment may be written  CSS=No Protection (other than CWRP)  AIVTDIS=Disabled AIVT  BSLIM=Not used  WDTEN=Disable  BTSWP=BOOTSWP instruction is disabled  DBCC=No Cross Connection between DAC outputs  CTXT1=Not Assigned  CTXT2=Not Assigned  SEQNUM=Not used  nSEQNUM=Not used  BOREN0=Enabled  DMTIVT=Not used  DMTCNT=2^31 (2147483648)  DMTEN=Dead Man Timer is Disabled and can be enabled by software  ON=Not used  USERID=Not used  RESERVED1=Not used  PGL1WAY=Allow only one reconfiguration  FPLLRNG=34-68 MHz Input  FPLLICLK=FRC is input to the System PLL  FPLLMULT=PLL Multiply by 128  UPLLFSEL=USB PLL input is 24 MHz  DMTINTV=Window/Interval value is 127/128 counter value  WDTSPGM=WDT stops during Flash programming  FDMTEN=Deadman Timer is disabled  TRCEN=Trace features in the CPU are enabled  BOOTISA=Boot code and Exception code is MIPS32  FECCCON=ECC and Dynamic ECC are disabled (ECCCON bits are writable)  EXTDDRSIZE=Not used  FSLEEP=Flash is powered down when the device is in Sleep mode  DBGPER=Allow CPU access to all permission regions  EJTAGBEN=Normal EJTAG functionality  TSEQ=Not used  CSEQ=Not used  RWDTPS=1:1048576  RCLKSEL=Always use LPRC  SWDTPS=1:1048576  DMTIVTL=Not used  DMTIVTH=Not used  DMTCNTL=Not used  DMTCNTH=Not used  DMTDIS=Dead Man Timer is Disabled and can be enabled by software  SMBEN=SMBus input threshold is enabled  SPI2PIN=SPI2 uses I/O remap (PPS) pins  CTXT3=Not Assigned  CTXT4=Not Assigned  MBXM0=Mailbox register configured for Master data read (Slave to Master data transfer)  MBXM1=Mailbox register configured for Master data read (Slave to Master data transfer)  MBXM2=Mailbox register configured for Master data read (Slave to Master data transfer)  MBXM3=Mailbox register configured for Master data read (Slave to Master data transfer)  MBXM4=Mailbox register configured for Master data read (Slave to Master data transfer)  MBXM5=Mailbox register configured for Master data read (Slave to Master data transfer)  MBXM6=Mailbox register configured for Master data read (Slave to Master data transfer)  MBXM7=Mailbox register configured for Master data read (Slave to Master data transfer)  MBXM8=Mailbox register configured for Master data read (Slave to Master data transfer)  MBXM9=Mailbox register configured for Master data read (Slave to Master data transfer)  MBXM10=Mailbox register configured for Master data read (Slave to Master data transfer)  MBXM11=Mailbox register configured for Master data read (Slave to Master data transfer)  MBXM12=Mailbox register configured for Master data read (Slave to Master data transfer)  MBXM13=Mailbox register configured for Master data read (Slave to Master data transfer)  MBXM14=Mailbox register configured for Master data read (Slave to Master data transfer)  MBXM15=Mailbox register configured for Master data read (Slave to Master data transfer)  MBXHSA=MSIxMBXD15 assigned to mailbox handshake protocol block A  MBXHSB=MSIxMBXD15 assigned to mailbox handshake protocol block B  MBXHSC=MSIxMBXD15 assigned to mailbox handshake protocol block C  MBXHSD=MSIxMBXD15 assigned to mailbox handshake protocol block D  MBXHSE=MSIxMBXD15 assigned to mailbox handshake protocol block E  MBXHSF=MSIxMBXD15 assigned to mailbox handshake protocol block F  MBXHSG=MSIxMBXD15 assigned to mailbox handshake protocol block G  MBXHSH=MSIxMBXD15 assigned to mailbox handshake protocol block H  HSAEN=Mailbox data flow control handshake protocol block disabled  HSBEN=Mailbox data flow control handshake protocol block disabled  HSCEN=Mailbox data flow control handshake protocol block disabled  HSDEN=Mailbox data flow control handshake protocol block disabled  HSEEN=Mailbox data flow control handshake protocol block disabled  HSFEN=Mailbox data flow control handshake protocol block disabled  HSGEN=Mailbox data flow control handshake protocol block disabled  HSHEN=Mailbox data flow control handshake protocol block disabled  CPRA0=Main core owns pin  CPRA1=Main core owns pin  CPRA2=Main core owns pin  CPRA3=Main core owns pin  CPRA4=Main core owns pin  CPRB0=Main core owns pin  CPRB1=Main core owns pin  CPRB2=Main core owns pin  CPRB3=Main core owns pin  CPRB4=Main core owns pin  CPRB5=Main core owns pin  CPRB6=Main core owns pin  CPRB7=Main core owns pin  CPRB8=Main core owns pin  CPRB9=Main core owns pin  CPRB10=Main core owns pin  CPRB11=Main core owns pin  CPRB12=Main core owns pin  CPRB13=Main core owns pin  CPRB14=Main core owns pin  CPRB15=Main core owns pin  CPRC0=Main core owns pin  CPRC1=Main core owns pin  CPRC2=Main core owns pin  CPRC3=Main core owns pin  CPRC4=Main core owns pin  CPRC5=Main core owns pin  CPRC6=Main core owns pin  CPRC7=Main core owns pin  CPRC8=Main core owns pin  CPRC9=Main core owns pin  CPRC10=Main core owns pin  CPRC11=Main core owns pin  CPRC12=Main core owns pin  CPRC13=Main core owns pin  CPRC14=Main core owns pin  CPRC15=Main core owns pin  CPRD0=Main core owns pin  CPRD1=Main core owns pin  CPRD2=Main core owns pin  CPRD3=Main core owns pin  CPRD4=Main core owns pin  CPRD5=Main core owns pin  CPRD6=Main core owns pin  CPRD7=Main core owns pin  CPRD8=Main core owns pin  CPRD9=Main core owns pin  CPRD10=Main core owns pin  CPRD11=Main core owns pin  CPRD12=Main core owns pin  CPRD13=Main core owns pin  CPRD14=Main core owns pin  CPRD15=Main core owns pin  CPRE0=Main core owns pin  CPRE1=Main core owns pin  CPRE2=Main core owns pin  CPRE3=Main core owns pin  CPRE4=Main core owns pin  CPRE5=Main core owns pin  CPRE6=Main core owns pin  CPRE7=Main core owns pin  CPRE8=Main core owns pin  CPRE9=Main core owns pin  CPRE10=Main core owns pin  CPRE11=Main core owns pin  CPRE12=Main core owns pin  CPRE13=Main core owns pin  CPRE14=Main core owns pin  CPRE15=Main core owns pin  S1FNOSC=Internal Fast RC (FRC) Oscillator with postscaler  S1IESO=Start up with FRC; then switch  S1OSCIOFNC=OSC2 is clock output  S1FCKSM=Both Clock switching and Fail-safe Clock Monitor are disabled  S1PLLKEN=S1PLLKEN_ON  S1RWDTPS=1:1048576  S1RCLKSEL=Always use LPRC  S1WINDIS=Watchdog Timer operates in Non-Window mode  S1WDTWIN=WDT Window is 25% of WDT period  S1SWDTPS=1:1048576  S1FWDTEN=use WDTCON.ON bit  S1ICS=Communicate on PGC3 and PGD3  S1DEBUG=Not used  S1ISOLAT=The slave can operate (in debug mode) even if the SLVEN bit in the MSI is zero  S1NOBTSWP=BOOTSWP instruction is disabled  S1ALTI2C1=I2C1 mapped to SDA1/SCL1 pins  S1SPI1PIN=Secondary SPI1 uses I/O remap (PPS) pins  S1SSRE=Slave generated resets will reset the Slave Enable Bit in the MSI module  S1MSRE=The master software oriented RESET events (RESET Op-Code; Watchdog timeout; TRAP reset; illegalInstruction) will also cause the slave subsystem to reset  S1CTXT1=Not Assigned  S1CTXT2=Not Assigned  S1CTXT3=Not Assigned  S1CTXT4=Not Assigned  BORLVL=BOR trip point is 2.96 V  BSSO=Normal startup operation after reset; execute instruction at 0x000000  MCA=Flash read accesses are 3 cycle (max frequency)  MAXTEMP=20 ns flash access  CFGAN14=Device pin is input to AN14  CFGAN15=Device pin is input to AN15  S1IOL1WAY=Allow only one reconfiguration  S1BSSO=Normal startup operation after reset; execute instruction at 0x000000  S1BACKBUG=Not used  BISTDIS=mBIST on reset feature disabled  NOBTSWP=BOOTSWP instruction is disabled  S1BISTDIS=Secondary BIST on reset feature disabled  S1DMTIVTL=Not used  S1DMTIVTH=Not used  S1DMTCNTL=Not used  S1DMTCNTH=Not used  S1DMTDIS=Secondary Dead Man Timer is Disabled and can be enabled by software  BSEQ=Not used  IBSEQ=Not used  SMB3EN=SMBus 3.0 input levels  FUSBIDIO2=USBID pin is controlled by the USB2 module  FVBUSIO2=VBUSON pin is controlled by the USB2 module  FUSBIDIO1=USBID pin is controlled by the USB1 module  FVBUSIO1=VBUSON pin is controlled by the USB1 module  VBATBOREN=Enable ZPBOR during VBAT Mode  FDSEN=Enable DSEN bit in DSCON  BORSEL=BOR trip voltage 2.1v (Non-OPAMP deviced operation)  POSCFGAIN=Gain is G3  POSCAGCDLY=Settling time = 25ms x AGCRNG  POSCAGCRNG=Range 1x  POSCAGC=Automatic Gain Control for Oscillator  FDBGWP=Not used
      settings: SourceProductName=MPLAB Device Blocks for Simulink
  Model Info : simulink/Model-Wide Utilities/Model Info  Frame=on  DisplayStringWithTags=|  HorizontalTextAlignment=Left  LeftAlignmentValue=0.02
      | Long hust motor with:
      | PHA - White
      | PHB - Black
      | PHC - Red
      | 
      | Encoder with:
      | QEA: Blue wire
      | QEB: White wire
      | +5V : Red wire
      | GND: Black wire
  Op-Amp : MCHP_Blockset/Analog IO/Op-Amp  Priority=-2000  OpAmp1=Enabled with positive and negative inputs  OpAmp2=Enabled with positive and negative inputs  OpAmp3=Disabled  S_INPUT=[-1]  S_INPUT_Size=[3]  S_OUTPUT=[]  S_OUTPUT_Size=[]  S_ListCustomDatatype=S.S_ListCustomDatatype={};  MCHP_USER_INTERRUPTS=0  MCHP_PORT={OA1 Output}{OA1out}14:2:A0;{OA1 IN+}{OA1in+}14:2:A2;{OA1 IN-}{OA1in-}14:2:A1;{OA2 Output}{OA2out}14:2:B2;{OA2 IN+}{OA2in+}14:2:B4;{OA2 IN-}{OA2in-}14:2:B3;  MCHP_MASTERLINK=mcb_pmsm_sixstep_hall_dsPIC33CK256MP508/Hardware Init/Microchip Master  MCHP_CRC=585153
      settings: SourceProductName=MPLAB Device Blocks for Simulink
  Open Board and Motor pages : Subsystem
      settings: OpenFcn=|
      | web('www.microchip.com/DevelopmentTools/ProductDetails.aspx?PartNO=DM330021-2','-browser');
      | pause(1);
      | web('http://www.microchipdirect.com/productsearch.aspx?keywords=AC300020','-browser');
      | pause(1);
      | web('www.microchipdirect.com/ProductSearch.aspx?keywords=AC300022','-browser');
      mask Display: disp('Open tools\nWebpage');
  Port Info : MCHP_Blockset/System Info/Port Info  MCHP_MASTERLINK=mcb_pmsm_sixstep_hall_dsPIC33CK256MP508/Hardware Init/Microchip Master
      settings: SourceProductName=MPLAB Device Blocks for Simulink
  Tasks State Show base rate Task on pin D8 (PIM) : MCHP_Blockset/Profiling/Tasks State  TasksPin=D8  MCHP_PORT={Task D1 Running}{Task D1}15:1:D8;  MCHP_MASTERLINK=mcb_pmsm_sixstep_hall_dsPIC33CK256MP508/Hardware Init/Microchip Master
      settings: SourceProductName=MPLAB Device Blocks for Simulink
  Timer Info : MCHP_Blockset/System Info/Timer Info  MCHP_MASTERLINK=mcb_pmsm_sixstep_hall_dsPIC33CK256MP508/Hardware Init/Microchip Master
      settings: SourceProductName=MPLAB Device Blocks for Simulink
  UART Configuration : MCHP_Blockset/BUS UART/UART Configuration  UART_REF=1  BAUD_Choice=Dynamic Options  BAUD_Choice_TXT="921600         [+0.01%]"  BAUD_Choice_IR=Dynamic Options  BAUD_Choice_IR_TXT=[]  BAUD_Custom=115200  INT_PRIORITY=0  ALT_IO=on  PIN_RX=Dynamic Options  PIN_RX_TXT=C9 / P57 / Pin[47]  PIN_TX=Dynamic Options  PIN_TX_TXT=D13 / P77 / Pin[14]  MCHP_PORT="{UART1  Tx}{U1TX}3:1:P77;"  MCHP_MASTERLINK=mcb_pmsm_sixstep_hall_dsPIC33CK256MP508/Hardware Init/Microchip Master  MCHP_COM_ExtPil=off  TX_IMPLEMENTATION=Circular Buffer  TX_IMPLEMENTATION_default=Circular Buffer  TX_INT_PRIORITY=5  TX_INT_WHEN=is empty & last char is sent  TX_INT_WHEN_default=is empty & last char is sent  TX_CIRCULAR_SIZE=64  TX_DMA_CHANNEL="0   (Lowest Priority)"  TX_DMA_SIZE=[]  TX_TASK_PROTECTION=Delay tasks (default)  TX_INTERRUPT_PROTECTION=Do not send on conflict (default)  TX_INTERRUPT_PROTECTION_default=Do not send on conflict (default)  RX_IMPLEMENTATION=Do not implement Rx  RX_IMPLEMENTATION_default=Circular Buffer  RX_INT_PRIORITY=5  RX_INT_WHEN=receive 1 character  RX_CIRCULAR_SIZE=128  RX_DMA_CHANNEL=0  RX_DMA_SIZE=0  DuplexMode=Full duplex (default)  PIN_RX_Inv=off  PIN_TX_Inv=off  PIN_RXTX_Inv=off  ParityBit=No parity (default)  StopBit=1 stop bit (default)  IRDA=off  FlowControl=None  PIN_CTS=Dynamic Options  PIN_CTS_TXT=B0 / P32 / Pin[34]  PIN_RTS=Dynamic Options  PIN_RTS_TXT=B0 / P32 / Pin[34]  InitSequence_chkbox=off  BAUD_Choice_InitSeq=Dynamic Options  BAUD_Choice_InitSeq_TXT="110         [+73.40%]"  BAUD_Choice_IR_InitSeq=Dynamic Options  BAUD_Choice_IR_InitSeq_TXT=0  BAUD_Custom_InitSeq=0  InitSequence='Hello World'
      settings: SourceProductName=MPLAB Device Blocks for Simulink

== system mcb_pmsm_sixstep_hall_dsPIC33CK256MP508/Heartbeat LED ==
  Counter Free-Running : simulink/Sources/Counter Free-Running  NumBits=1  tsamp=0.5
  Counter Free-Running1 : simulink/Sources/Counter Free-Running  NumBits=1  tsamp=0.1
  Data Type Conversion : DataTypeConversion  OutDataTypeStr=boolean  SaturateOnIntegerOverflow=off  RndMeth=Floor
  Data Type Conversion1 : DataTypeConversion  OutDataTypeStr=boolean  SaturateOnIntegerOverflow=off  RndMeth=Floor
  LED 1 : MCHP_Blockset/Digital IO/Digital Output  PORT=Dynamic Options  PORT_TXT="E   [ 0 : 15 ]"  PIN=6  PACK=off  SIMULTANEOUS=off  READPREVIOUS=off  ORDERING=None  SampleTime=-1  MCHP_MASTERLINK=mcb_pmsm_sixstep_hall_dsPIC33CK256MP508/Hardware Init/Microchip Master
      settings: SourceProductName=MPLAB Device Blocks for Simulink
  LED 2 : MCHP_Blockset/Digital IO/Digital Output  PORT=Dynamic Options  PORT_TXT="E   [ 0 : 15 ]"  PIN=7  PACK=off  SIMULTANEOUS=off  READPREVIOUS=off  ORDERING=None  SampleTime=-1  MCHP_MASTERLINK=mcb_pmsm_sixstep_hall_dsPIC33CK256MP508/Hardware Init/Microchip Master
      settings: SourceProductName=MPLAB Device Blocks for Simulink
  wires:
  Data Type Conversion/1 -> LED 1/1
  Counter Free-Running/1 -> Data Type Conversion/1
  Counter Free-Running1/1 -> Data Type Conversion1/1
  Data Type Conversion1/1 -> LED 2/1

== system mcb_pmsm_sixstep_hall_dsPIC33CK256MP508/Inverter and Motor ==
  Duty_Cycles_hall : Inport
  Codegeneration : Subsystem
  Simulation : Subsystem
  Variant Sink1 : VariantSink
  Variant Source2 : VariantSource
  Feedbacks_hall : Outport  VectorParamsAs1DForOutWhenUnconnected=off
  wires:
  Simulation/1(Hall_fb) -> Variant Source2/2
  Codegeneration/1(fb_codegen) -> Variant Source2/1
  Variant Source2/1 -> Feedbacks_hall/1
  Duty_Cycles_hall/1 -> Variant Sink1/1
  Variant Sink1/1 -> Codegeneration/1(Duty_Cycles_Hall)
  Variant Sink1/2 -> Simulation/1(Duty_Cycles_Hall)

== system mcb_pmsm_sixstep_hall_dsPIC33CK256MP508/Speed Control ==
  Speed_Ref_PU : Inport
  Speed_Meas_PU : Inport  Port=2
  Data Store Write : DataStoreWrite  DataStoreName=Speed_ref  IndexOptions=Index vector (dialog)  Indices=1  OutputSizes=1
  Data Type Conversion : DataTypeConversion  SaturateOnIntegerOverflow=off  RndMeth=Floor
  PI_Controller_Speed : Subsystem
  Saturation : Saturate  UpperLimit=(bldc.N_max/bldc.N_base)  LowerLimit=(300/bldc.N_base)
  Speed_Ref_Selector : Subsystem
  Step : Step  Time=3  Before=0.2  After=0.7
  Variant Source1 : VariantSource
  Duty_PU : Outport  VectorParamsAs1DForOutWhenUnconnected=off
  wires:
  Speed_Meas_PU/1 -> PI_Controller_Speed/2(N_fb)  "Speed_fb"
  Speed_Ref_Selector/1(Speed_Ref_PU) -> Data Store Write/1, PI_Controller_Speed/1(N_ref)  "Speed_Ref"
  PI_Controller_Speed/1(Iq_ref) -> Duty_PU/1
  Saturation/1 -> Speed_Ref_Selector/1(Speed_Ref_In)
  Variant Source1/1 -> Saturation/1
  Speed_Ref_PU/1 -> Variant Source1/1
  Step/1 -> Data Type Conversion/1
  Data Type Conversion/1 -> Variant Source1/2

== system mcb_pmsm_sixstep_hall_dsPIC33CK256MP508/Current Control/Input Scaling ==
  Hall : Inport
  Hall_Sim : Inport  Port=2
  Hall Feedback : Subsystem  TreatAsAtomicUnit=on
  Subsystem : Subsystem
  Variant Source1 : VariantSource
  Variant Source3 : VariantSource
  Hall_State : Outport
  Speed_PU : Outport  Port=2
  wires:
  Hall Feedback/1(HallState) -> Variant Source3/2
  Hall_Sim/1 -> Hall Feedback/1(Hall_Meas)
  Variant Source3/1 -> Hall_State/1
  Hall/1 -> Subsystem/1(Hall_State)
  Subsystem/1(HallState) -> Variant Source3/1
  Subsystem/2(Speed_PU) -> Variant Source1/1
  Hall Feedback/2(Speed_PU) -> Variant Source1/2
  Variant Source1/1 -> Speed_PU/1

== system mcb_pmsm_sixstep_hall_dsPIC33CK256MP508/Current Control/MOTOR Cmd ==
  PWM (abc) : Inport
  Dead time Compensation : Bias  Bias=round( (inverter.deadtime/5e-5) *PWM1max )  SaturateOnIntegerOverflow=off
  Demux : Demux  Outputs=3
  PWM_HS_FEP : MCHP_Blockset/PWM IO/PWM_HS_FEP  Priority=-2000  PWMx_MODSEL=Center Aligned  PWMx_CLKSEL=no scaling  PWM_ClockResolution_DIVSEL=Dynamic Options  PWM_ClockResolution_DIVSEL_TXT=auto  PWM_ClockResolution_FSCL=Dynamic Options  PWM_ClockResolution_FSCL_TXT=auto - no jitter  PWM_ClockResolution_NoScaling=Dynamic Options  PWM_ClockResolution_NoScaling_TXT="Resol: 0.005(us)  -  MaxPer: 0.000328(s)"  MaxPeriod_s=50e-6  InitPeriode_s=50e-6  InitDutyCycleP_s=2e-6  InitDutyCycleS_s=10e-6  InitPhase_s=-1  evalin_ws=PWM1max=MCHP_Fun.Hex2num('40B3880000000000');PWM2max=MCHP_Fun.Hex2num('40B3880000000000');PWM4max=MCHP_Fun.Hex2num('40B3880000000000');  SampleTime=Ts  S_INPUT=[-1]  S_INPUT_Size=[3]  S_OUTPUT=[]  S_OUTPUT_Size=[]  S_ListCustomDatatype=S.S_ListCustomDatatype={};  MCHP_USER_INTERRUPTS=0  MCHP_PORT={PWMH1 }{PWMH1}32:4:B14;{PWMH2 }{PWMH2}32:4:B12;{PWMH4 }{PWMH4}32:4:D1;{PWML1}{PWML1}32:4:B15;{PWML2}{PWML2}32:4:B13;{PWML4}{PWML4}32:4:D0;  MCHP_MASTERLINK=mcb_pmsm_sixstep_hall_dsPIC33CK256MP508/Hardware Init/Microchip Master  MCHP_CRC=4912622  PWMx_PMOD=Complementary  PWM1_HL=PWMxH & PWMxL output enabled  PWM1_swap=off  PWM1H_pol=off  PWM1L_pol=off  PWM2_HL=PWMxH & PWMxL output enabled  PWM2_swap=off  PWM2H_pol=off  PWM2L_pol=off  PWM3_HL=not used  PWM3_swap=off  PWM3H_pol=off  PWM3L_pol=off  PWM4_HL=PWMxH & PWMxL output enabled  PWM4_swap=off  PWM4H_pol=off  PWM4L_pol=off  PWM5_HL=not used  PWM5_swap=off  PWM5H_pol=off  PWM5L_pol=off  PWM6_HL=not used  PWM6_swap=off  PWM6H_pol=off  PWM6L_pol=off  PWM7_HL=not used  PWM7_swap=off  PWM7H_pol=off  PWM7L_pol=off  PWM8_HL=not used  PWM8_swap=off  PWM8H_pol=off  PWM8L_pol=off  PWM9_HL=not used  PWM9_swap=off  PWM9H_pol=off  PWM9L_pol=off  PWM10_HL=not used  PWM10_swap=off  PWM10H_pol=off  PWM10L_pol=off  PWM11_HL=not used  PWM11_swap=off  PWM11H_pol=off  PWM11L_pol=off  PWM12_HL=not used  PWM12_swap=off  PWM12H_pol=off  PWM12L_pol=off  PWM1_ShowTrig=on  PWM1_Init_PGxTRIGABC_s=[0 -1 -1 ]  PWM1_ADTRxEN1=ADC Trigger 1  PWM1_ADTRxEN2=none  PWM1_ADTRxEN3=none  PWM2_ShowTrig=off  PWM2_Init_PGxTRIGABC_s=[-1 -1 -1]  PWM2_ADTRxEN1=none  PWM2_ADTRxEN2=none  PWM2_ADTRxEN3=none  PWM3_ShowTrig=off  PWM3_Init_PGxTRIGABC_s=[-1 -1 -1]  PWM3_ADTRxEN1=none  PWM3_ADTRxEN2=none  PWM3_ADTRxEN3=none  PWM4_ShowTrig=off  PWM4_Init_PGxTRIGABC_s=[-1 -1 -1]  PWM4_ADTRxEN1=none  PWM4_ADTRxEN2=none  PWM4_ADTRxEN3=none  PWM5_ShowTrig=off  PWM5_Init_PGxTRIGABC_s=[-1 -1 -1]  PWM5_ADTRxEN1=none  PWM5_ADTRxEN2=none  PWM5_ADTRxEN3=none  PWM6_ShowTrig=off  PWM6_Init_PGxTRIGABC_s=[-1 -1 -1]  PWM6_ADTRxEN1=none  PWM6_ADTRxEN2=none  PWM6_ADTRxEN3=none  PWM7_ShowTrig=off  PWM7_Init_PGxTRIGABC_s=[-1 -1 -1]  PWM7_ADTRxEN1=none  PWM7_ADTRxEN2=none  PWM7_ADTRxEN3=none  PWM8_ShowTrig=off  PWM8_Init_PGxTRIGABC_s=[-1 -1 -1]  PWM8_ADTRxEN1=none  PWM8_ADTRxEN2=none  PWM8_ADTRxEN3=none  BlockInput_VectorScalar=Independant Scalar  BlockInput_Period=Not a block input  BlockInput_DutyCycle=a Uint raw input (PWMxmax variable represent max period)  BlockInput_PhaseShift=Not a block input  BlockInput_SEVTCMP=Not a block input  BlockInput_TRIGx=Not a block input  BlockInput_DeadTime=Not a block input  BlockOutput_FaultDisabled=off  BlockOutput_Fault=on  DTC=Positive dead time (ensure period of time with PWM_H and PWM_L disasserted)  FLTSRC1_DTCMP=Dynamic Options  FLTSRC1_DTCMP_TXT=<empty>  FLTSRC2_DTCMP=Dynamic Options  FLTSRC2_DTCMP_TXT=<empty>  FLTSRC3_DTCMP=Dynamic Options  FLTSRC3_DTCMP_TXT=<empty>  FLTSRC4_DTCMP=Dynamic Options  FLTSRC4_DTCMP_TXT=<empty>  FLTSRC5_DTCMP=Dynamic Options  FLTSRC5_DTCMP_TXT=<empty>  FLTSRC6_DTCMP=Dynamic Options  FLTSRC6_DTCMP_TXT=<empty>  FLTSRC7_DTCMP=Dynamic Options  FLTSRC7_DTCMP_TXT=<empty>  FLTSRC8_DTCMP=Dynamic Options  FLTSRC8_DTCMP_TXT=<empty>  FLTSRC9_DTCMP=Dynamic Options  FLTSRC9_DTCMP_TXT=<empty>  FLTSRC10_DTCMP=Dynamic Options  FLTSRC10_DTCMP_TXT=<empty>  FLTSRC11_DTCMP=Dynamic Options  FLTSRC11_DTCMP_TXT=<empty>  FLTSRC12_DTCMP=Dynamic Options  FLTSRC12_DTCMP_TXT=<empty>  DeadTime_s=2e-6  DeadTimeAlt_s=2e-6  DeadTimeComp_s=0  FLTMODx=Disabled  FLTSRCx=Dynamic Options  FLTSRCx_TXT=<empty>  FLTDATx=PWM H/L -> 11  CLMODx=Disabled  CLSRCx=Dynamic Options  CLSRCx_TXT=<empty>  CLDATx=PWM H/L -> 00  FLTLEBENx=off  CLLEBENx=off  LeadEdgeBlkPer_s=5e-7  PHRx=off  PHFx=off  PLRx=off  PLFx=off
      settings: SourceProductName=MPLAB Device Blocks for Simulink
  "Saturation " : Saturate  UpperLimit=PWM1max  LowerLimit=round( (inverter.deadtime/5e-5) *PWM1max )* 2
  int to uint : DataTypeConversion  OutDataTypeStr=uint16  ConvertRealWorld=Stored Integer (SI)  SaturateOnIntegerOverflow=off  RndMeth=Floor
  wires:
  int to uint/1 -> "Saturation "/1
  Dead time Compensation/1 -> int to uint/1
  PWM (abc)/1 -> Dead time Compensation/1
  "Saturation "/1 -> Demux/1
  Demux/2 -> PWM_HS_FEP/2
  Demux/3 -> PWM_HS_FEP/3
  Demux/1 -> PWM_HS_FEP/1
